simulink model "exp4_storageTank_varianceTimeConstant_Gain"  (R2023a)
settings: Solver=VariableStepAuto  StartTime=0.0  StopTime=10.0  FixedStep=0.1  RelTol=1e-3
settings Model: Creator=nipun  LastModifiedBy=nipun

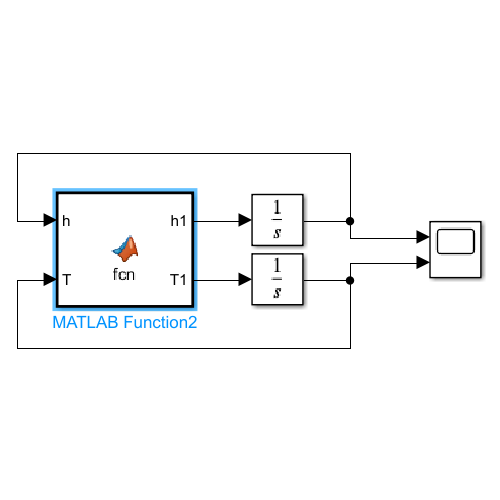
[thumbnail: Simulink's stored preview of the top-level diagram]
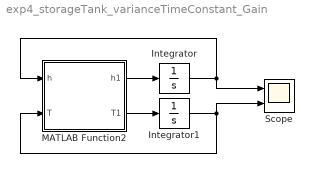
== system exp4_storageTank_varianceTimeConstant_Gain ==
  Integrator : Integrator
  Integrator1 : Integrator
  MATLAB Function2 : MATLAB Function  TreatAsAtomicUnit=on
  Scope : Scope  NumInputPorts=2
  wires:
  MATLAB Function2/1(h1) -> Integrator/1
  Integrator/1 -> MATLAB Function2/1(h), Scope/1
  MATLAB Function2/2(T1) -> Integrator1/1
  Integrator1/1 -> MATLAB Function2/2(T), Scope/2

== matlab function exp4_storageTank_varianceTimeConstant_Gain/MATLAB Function2 ==
  data: h1 output; h input; T1 output; T input
function [h1,T1] = fcn(h,T)
A=1;
pho=1;
B=1;
Cp=1;
Q=1;
Ti=29;
Fi=1;
Fo=B*sqrt(h);
h1=(Fi-Fo)/(A);
disp(h);
if(h<1e-2)
    T1=0;
else
    T1=(Fi*(Ti-T)+Q/(pho*Cp))/(A*h);
end
disp(T1);
